simulink model "double_buf"  (R2012b)
settings: Solver=ode45  StartTime=0.0  StopTime=10.0  RelTol=1e-3
libraries: xbsIndex_r4 x5
settings Model: Creator=jack  LastModifiedBy=jack

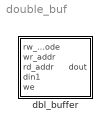
== system double_buf ==
  dbl_buffer : Subsystem  AncestorBlock=casper_library_reorder/dbl_buffer  mask(dbl_buffer){depth=32, latency=2}

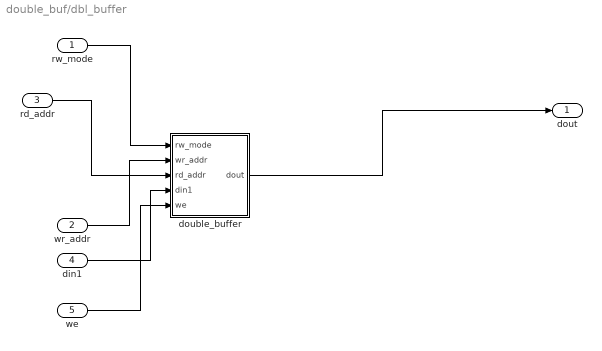
== system double_buf/dbl_buffer ==
  rw_mode : Inport
  wr_addr : Inport  Port=2
  rd_addr : Inport  Port=3
  din1 : Inport  Port=4
  we : Inport  Port=5
  double_buffer : Subsystem
  dout : Outport
  wires:
  rw_mode/1 -> double_buffer/1(rw_mode)
  wr_addr/1 -> double_buffer/2(wr_addr)
  rd_addr/1 -> double_buffer/3(rd_addr)
  din1/1 -> double_buffer/4(din1)
  we/1 -> double_buffer/5(we)
  double_buffer/1(dout) -> dout/1

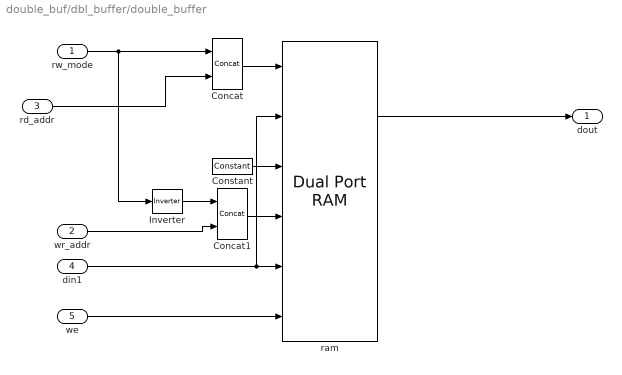
== system double_buf/dbl_buffer/double_buffer ==
  rw_mode : Inport
  wr_addr : Inport  Port=2
  rd_addr : Inport  Port=3
  din1 : Inport  Port=4
  we : Inport  Port=5
  Concat : xbsIndex_r4/Concat  num_inputs=2  dbl_ovrd=off  block_type=concat
  Concat1 : xbsIndex_r4/Concat  num_inputs=2  dbl_ovrd=off  block_type=concat
  Constant : xbsIndex_r4/Constant  const=0  gui_display_data_type=Fixed-point  arith_type=Boolean  n_bits=1  bin_pt=0  preci_type=Single  exp_width=8  frac_width=24  explicit_period=on  period=1  equ=P=C  opselect=C  inp2=PCIN>>17  opr=+  inp1=P  carry=CIN  dbl_ovrd=off  block_type=constant
      settings: block_version=9.1.01
  Inverter : xbsIndex_r4/Inverter  en=off  latency=0  dbl_ovrd=off  block_type=inv
  ram : xbsIndex_r4/Dual Port RAM  depth=1024  initVector=0  distributed_mem=Block RAM  init_a=0  init_b=0  rst_a=off  rst_b=off  en_a=off  en_b=off  latency=3  write_mode_A=Read Before Write  write_mode_B=No Read On Write  dbl_ovrd=off  optimize=Speed  block_type=dpram
  dout : Outport
  wires:
  ram/1 -> dout/1
  we/1 -> ram/6
  din1/1 -> ram/2, ram/5
  Constant/1 -> ram/3
  rd_addr/1 -> Concat/2
  rw_mode/1 -> Inverter/1, Concat/1
  Concat/1 -> ram/1
  wr_addr/1 -> Concat1/2
  Concat1/1 -> ram/4
  Inverter/1 -> Concat1/1
